simulink model "ExampleTyre"  (Simulink 9.2)
settings: Solver=ode1  StartTime=0.0  StopTime=10.0  FixedStep=0.0025  RelTol=1e-3  EnableMultiTasking=on
libraries: rFproPhysicsLib x4, simulink x1
Description:
  | Compiled Plugin Only
settings Model: Creator=enewton  LastModifiedBy=SeanKavanagh
settings OptimizationCC: ExpressionDepthLimit=2147483647
settings DebuggingCC: SolverPrmCheckMsg=warning  InheritedTsInSrcMsg=none
settings RTWCC: SystemTargetFile=rfpro.tlc  MakeCommand="make_rtw OPTS=\"-DCOMPUTE_TYRE\""  TemplateMakefile=rfpro.tmf  Description=rFactor Pro Target (Compute ISO Tyre Forces)  TargetLang=C++
settings STFCustomTargetCC: ModelReferenceCompliant=off  GeneratePreprocessorConditionals=Disable all  CombineOutputUpdateFcns=on  MatFileLogging=on  CPPClassGenCompliant=on  GRTInterface=off  SystemTargetFile=rfpro.tlc
settings GRTTargetCC: ModelReferenceCompliant=off  ParMdlRefBuildCompliant=off  CompOptLevelCompliant=off  ConcurrentExecutionCompliant=off  CombineOutputUpdateFcns=on  GRTInterface=off  UseToolchainInfoCompliant=off  ExtModeMexFile=noextcomm

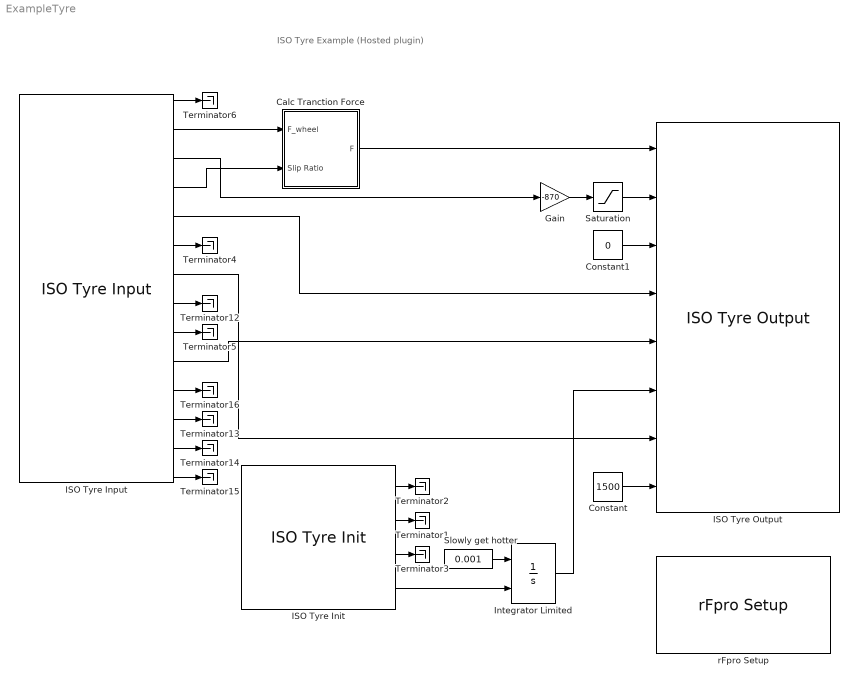
== system ExampleTyre ==
  note: ISO Tyre Example (Hosted plugin)
  Calc Tranction Force : Subsystem
  Constant : Constant  Value=1500
  Constant1 : Constant  Value=0
  Gain : Gain  Gain=-870
  ISO Tyre Init : rFproPhysicsLib/Hosted Blocks/ISO Tyre Init  SFunctionModules=''
  ISO Tyre Input : rFproPhysicsLib/Hosted Blocks/ISO Tyre Input  SFunctionModules=''
  ISO Tyre Output : rFproPhysicsLib/Hosted Blocks/ISO Tyre Output  SFunctionModules=''
  Integrator Limited : Integrator  InitialConditionSource=external  LimitOutput=on  UpperSaturationLimit=1000  LowerSaturationLimit=-200
  Saturation : Saturate  UpperLimit=5000  LowerLimit=-5000
  Slowly get hotter : Constant  Value=0.001
  Terminator{1..6,12..16} (11 alike) : Terminator
  rFpro Setup : rFproPhysicsLib/rFpro Setup  Priority=1  platform=Hosted Plugin  stopOnSessionEnd=on  usePseudoRealtime=on  syncToRF=on  useReverseByteOrder=off  useRfTime=on  minIterations=4  maxIterations=1000  ipReceiveAddress='127.0.0.1'  ipReceivePort=11054  receiveSampleTime=-1  ipTransmitAddress='127.0.0.1'  ipTransmitPort=11052  transmitSampleTime=-1  pluginType=COMPUTE_TYRE
  wires:
  Integrator Limited/1 -> ISO Tyre Output/6
  ISO Tyre Init/4 -> Integrator Limited/2
  Slowly get hotter/1 -> Integrator Limited/1
  ISO Tyre Init/1 -> Terminator2/1
  ISO Tyre Init/2 -> Terminator1/1
  ISO Tyre Init/3 -> Terminator3/1
  ISO Tyre Input/1 -> Terminator6/1
  ISO Tyre Input/2 -> Calc Tranction Force/1(F_wheel)
  ISO Tyre Input/3 -> Gain/1
  ISO Tyre Input/4 -> Calc Tranction Force/2(Slip Ratio)
  ISO Tyre Input/8 -> Terminator12/1
  ISO Tyre Input/11 -> Terminator16/1
  ISO Tyre Input/13 -> Terminator14/1
  ISO Tyre Input/14 -> Terminator15/1
  Constant/1 -> ISO Tyre Output/8
  Constant1/1 -> ISO Tyre Output/3
  ISO Tyre Input/5 -> ISO Tyre Output/4
  ISO Tyre Input/10 -> ISO Tyre Output/5
  ISO Tyre Input/12 -> Terminator13/1
  ISO Tyre Input/7 -> ISO Tyre Output/7
  Calc Tranction Force/1(F) -> ISO Tyre Output/1
  ISO Tyre Input/9 -> Terminator5/1
  ISO Tyre Input/6 -> Terminator4/1
  Gain/1 -> Saturation/1
  Saturation/1 -> ISO Tyre Output/2

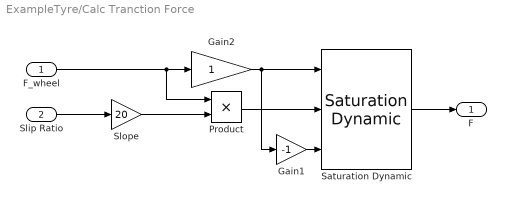
== system ExampleTyre/Calc Tranction Force ==
  F_wheel : Inport
  Slip Ratio : Inport  Port=2
  Gain1 : Gain  Gain=-1
  Gain2 : Gain
  Product : Product
  Saturation Dynamic : simulink/Discontinuities/Saturation Dynamic  OutMin=[]  OutMax=[]  OutDataTypeStr=Inherit: Same as second input  OutDataType=fixdt(1, 16)  OutScaling=2^-10  DoSatur=off
  Slope : Gain  Gain=20
  F : Outport
  wires:
  Slope/1 -> Product/2
  Gain1/1 -> Saturation Dynamic/3
  Saturation Dynamic/1 -> F/1
  Product/1 -> Saturation Dynamic/2
  F_wheel/1 -> Product/1, Gain2/1
  Gain2/1 -> Gain1/1, Saturation Dynamic/1
  Slip Ratio/1 -> Slope/1
